simulink model "sf_tlafter"  (Simulink 6.0)
settings: Solver=ode45  StartTime=0.0  StopTime=100  RelTol=1e-3
settings Model: CovMetricSettings=dcmtr  Creator=The MathWorks Inc.  LastModifiedBy=batserve  ExtModeAutoUpdateStatusClock=off
settings OptimizationCC: BooleanDataType=off
settings DebuggingCC: CheckExecutionContextPreStartOutputMsg=on  CheckExecutionContextRuntimeOutputMsg=on  SolverPrmCheckMsg=none
settings HardwareCC: TargetUnknown=on

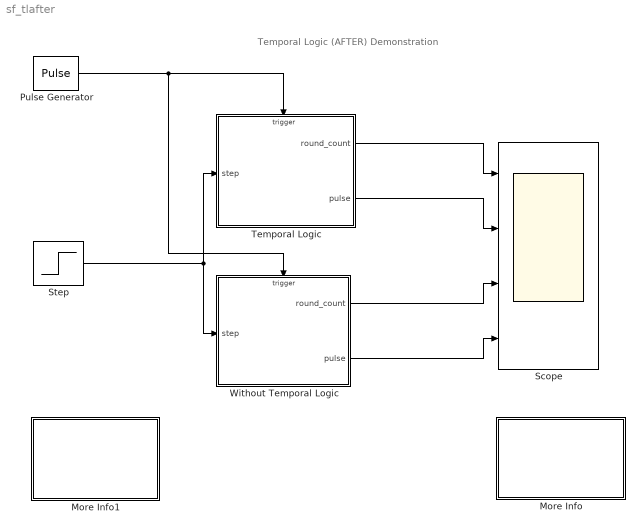
== system sf_tlafter ==
  note: Temporal Logic (AFTER) Demonstration
  More Info : Subsystem  PropExecContextAcrossSSBoundary=on
      mask Display: disp('Double click\nhere for\ninformation on\nthis demonstration')
  More Info1 : Subsystem  PropExecContextAcrossSSBoundary=on
      settings: OpenFcn=simcad(bdroot);
      mask Display: disp('Double click\nhere for\nSimulink\Stateflow\n Help')
  Pulse Generator : DiscretePulseGenerator  PulseType=Time based  Period=1  PulseWidth=50
  Scope : Scope  NumInputPorts=4
      settings: TimeRange=100  YMin=0~-0.5~0~-0.5  YMax=6~1.5~6~1.5
  Step : Step  Time=60  SampleTime=0
  Temporal Logic : Stateflow chart  TreatAsAtomicUnit=on  PropExecContextAcrossSSBoundary=on
  Without Temporal Logic : Stateflow chart  TreatAsAtomicUnit=on  PropExecContextAcrossSSBoundary=on
  wires:
  Pulse Generator/1 -> Temporal Logic/Trigger, Without Temporal Logic/Trigger
  Temporal Logic/1(round_count) -> Scope/1
  Temporal Logic/2(pulse) -> Scope/2
  Without Temporal Logic/1(round_count) -> Scope/3
  Without Temporal Logic/2(pulse) -> Scope/4
  Step/1 -> Temporal Logic/1(step), Without Temporal Logic/1(step)

== system sf_tlafter/More Info ==
  note: This simple demonstration compares the difference between two Stateflow charts: one chart
      | uses temporal logic and the AFTER function to achieve the goal, and the other chart achieves
      | the same goal without using temporal logic.
      |
      | The AFTER function allows you to easily obtain the number of events that have occurred within
      | that chart and then used as a condition for an event transition. For example, in this demonstration,
      | a transition from the 'Off' to the 'On' state will occur after 10 events (labeled as 'secs') have passed
      | as long as the input, 'step', is less than 1. In this case the input 'step' is created using a Step
      | function block from Simulink and the event 'secs' is defined by using a Pulse Generator. The value
      |  of this step will be zero until 60 seconds of simulation have gone by. After 60 seconds pass, the
      | step is created and the value of the step input is 1. Since one of the transition conditions in the
      | chart is not met ('step' < 1) then the transition does not take place anymore and you can notice a
      | halt in the chart activity.
      |
      | The same effect is achieved without the use of temporal logic. The difference is that an additional
      | variable and transition need to be included in order to count the number of times an event takes
      | place. In this case, the local variable 'count_after' is used to obtain the number of times the event
      | 'secs' occurs. The transition will then take place if 'count_after' is greater than 10 and the value of
      | step (which is the input) is less than 1.
  note: Temporal Logic using the AFTER function

== system sf_tlafter/More Info1 ==

== stateflow chart Temporal Logic ==
  state Off
  state On
    en:pulse=1;
    exit:pulse=0;
  Off -> On : after(10,secs)[step<1]
  On -> Off : {round_count++;}
  (default) -> Off : {round_count=0;}
  data: round_count output double; pulse output double; step input double
  events: secs input RISING_EDGE_EVENT

== stateflow chart Without Temporal Logic ==
  state On [parallel]
    state A
      count_after=2;
      A -> A : {count_after++;}
    state B
      entry: pulse=1;
      exit: pulse=0;
    A -> B : [count_after>10 && step<1]
    B -> A : {round_count++;}
  (default) -> A
  data: count local double; round_count output double; count_after local double; pulse output double; step input double
  events: secs input RISING_EDGE_EVENT
